simulink model "[LQG] Inverse_Pendulum_discretized"  (R2022b)
settings: Solver=ode4  StartTime=0.0  StopTime=50  FixedStep=0.005  RelTol=1e-3
values from neighbouring files (symbols this model uses):
  Ad = sys_d.A    [Inverse_Pendulum_parameters_discrete.m]
  b = 0.00007892    (= 7.892e-05)    [Inverse_Pendulum_parameters.m]    (also in Inverse_Pendulum_parameters_discrete.m; [LQG] Inverse_Pendulum_parameters.m; [LQR] Inverse_Pendulum_parameters.m)
  Bd = sys_d.B    [Inverse_Pendulum_parameters_discrete.m]
  c = 0.63    [Inverse_Pendulum_parameters.m]    (also in Inverse_Pendulum_parameters_discrete.m; [LQG] Inverse_Pendulum_parameters.m; [LQR] Inverse_Pendulum_parameters.m)
  Cd = sys_d.C    [Inverse_Pendulum_parameters_discrete.m]
  g = 9.81    [Inverse_Pendulum_parameters.m]    (also in Inverse_Pendulum_parameters_discrete.m; [LQG] Inverse_Pendulum_parameters.m; [LQR] Inverse_Pendulum_parameters.m)
  J = 0.0007176    [Inverse_Pendulum_parameters.m]    (also in Inverse_Pendulum_parameters_discrete.m = 0.000596; [LQG] Inverse_Pendulum_parameters.m; [LQR] Inverse_Pendulum_parameters.m)
  k_swing = 12    [Inverse_Pendulum_parameters.m]    (also in Inverse_Pendulum_parameters_discrete.m = 42; [LQG] Inverse_Pendulum_parameters.m; [LQR] Inverse_Pendulum_parameters.m)
  kb = 0.031    [Inverse_Pendulum_parameters.m]    (also in Inverse_Pendulum_parameters_discrete.m; [LQG] Inverse_Pendulum_parameters.m; [LQR] Inverse_Pendulum_parameters.m)
  Kd = dlqr(Ad, Bd, Q, R)    [Inverse_Pendulum_parameters_discrete.m]
  Kkd = dlqe(Ad, G, Cd, Qn, Rn)    [Inverse_Pendulum_parameters_discrete.m]
  kt = 0.031    [Inverse_Pendulum_parameters.m]    (also in Inverse_Pendulum_parameters_discrete.m; [LQG] Inverse_Pendulum_parameters.m; [LQR] Inverse_Pendulum_parameters.m)
  l = 0.2    [Inverse_Pendulum_parameters.m]    (also in Inverse_Pendulum_parameters_discrete.m = 0.1; [LQG] Inverse_Pendulum_parameters.m; [LQR] Inverse_Pendulum_parameters.m)
  M = 0.136    [Inverse_Pendulum_parameters.m]    (also in Inverse_Pendulum_parameters_discrete.m = 0.1; [LQG] Inverse_Pendulum_parameters.m; [LQR] Inverse_Pendulum_parameters.m)
  m = 0.1    [Inverse_Pendulum_parameters.m]    (also in Inverse_Pendulum_parameters_discrete.m = 0.04467; [LQG] Inverse_Pendulum_parameters.m; [LQR] Inverse_Pendulum_parameters.m)
  r = 0.006    [Inverse_Pendulum_parameters.m]    (also in Inverse_Pendulum_parameters_discrete.m; [LQG] Inverse_Pendulum_parameters.m; [LQR] Inverse_Pendulum_parameters.m)
  Rm = 12.5    [Inverse_Pendulum_parameters.m]    (also in Inverse_Pendulum_parameters_discrete.m; [LQG] Inverse_Pendulum_parameters.m; [LQR] Inverse_Pendulum_parameters.m)
  Ts = 0.005    [Inverse_Pendulum_parameters_discrete.m]
libraries: simulink x8, mpclib x2
settings Model: Creator=ADMIN  LastModifiedBy=ADMIN
settings OptimizationCC: DefaultParameterBehavior=Inlined  EnhancedBackFolding=on  PassReuseOutputArgsAs=Individual arguments  ZeroExternalMemoryAtStartup=off  ZeroInternalMemoryAtStartup=off  OptimizeBlockOrder=speed  DifferentSizesBufferReuse=on  OptimizationCustomize=off  EfficientTunableParamExpr=on
settings DebuggingCC: ParameterTunabilityLossMsg=error
settings SFSimCC: MATLABDynamicMemAlloc=off
settings RTWCC: Description=Embedded Coder  SystemTargetFile=ert.tlc  GenCodeOnly=on  TemplateMakefile=ert_default_tmf  GPUComputeCapability=5.0
settings CodeAppCC: ForceParamTrailComments=on  IgnoreCustomStorageClasses=off  OperatorAnnotations=on  SimulinkDataObjDesc=on  SFDataObjDesc=on  InsertBlockDesc=on
settings ERTTargetCC: TargetLangStandard=C99 (ISO)  GenerateSampleERTMain=on  InlinedParameterPlacement=NonHierarchical  ERTCustomFileTemplate=example_file_process.tlc

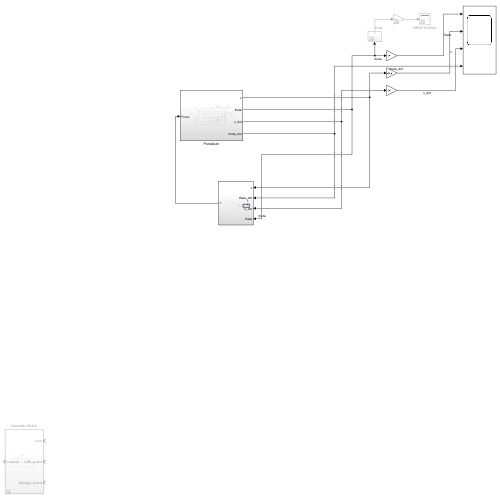
[thumbnail: Simulink's stored preview of the top-level diagram]
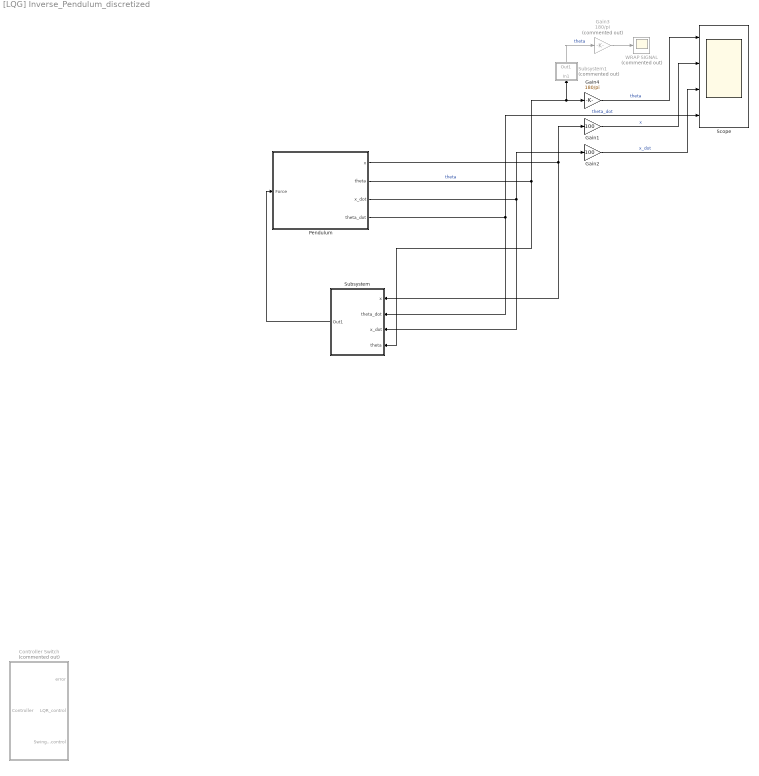
== system [LQG] Inverse_Pendulum_discretized ==
  Controller Switch : Subsystem  Commented=on
  Gain1 : Gain  Gain=100
  Gain2 : Gain  Gain=100
  Gain3 : Gain  Commented=on  Gain=180/pi
  Gain4 : Gain  Gain=180/pi
  Pendulum : Subsystem
  Scope : Scope  NumInputPorts=4
  Subsystem : Subsystem
  Subsystem1 : Subsystem  Commented=on
  WRAP SIGNAL : Scope  Commented=on
  wires:
  Pendulum/1(x) -> Gain1/1, Subsystem/1(x)
  Pendulum/3(x_dot) -> Gain2/1, Subsystem/3(x_dot)
  Pendulum/4(theta_dot) -> Scope/4, Subsystem/2(theta_dot)  "theta_dot"
  Gain1/1 -> Scope/2  "x"
  Gain2/1 -> Scope/3  "x_dot"
  Pendulum/2(theta) -> Subsystem/4(theta), Subsystem1/1(In1), Gain4/1  "theta"
  Gain3/1 -> WRAP SIGNAL/1
  Subsystem1/1(Out1) -> Gain3/1  "theta"
  Gain4/1 -> Scope/1  "theta"
  Subsystem/1(Out1) -> Pendulum/1(Force)

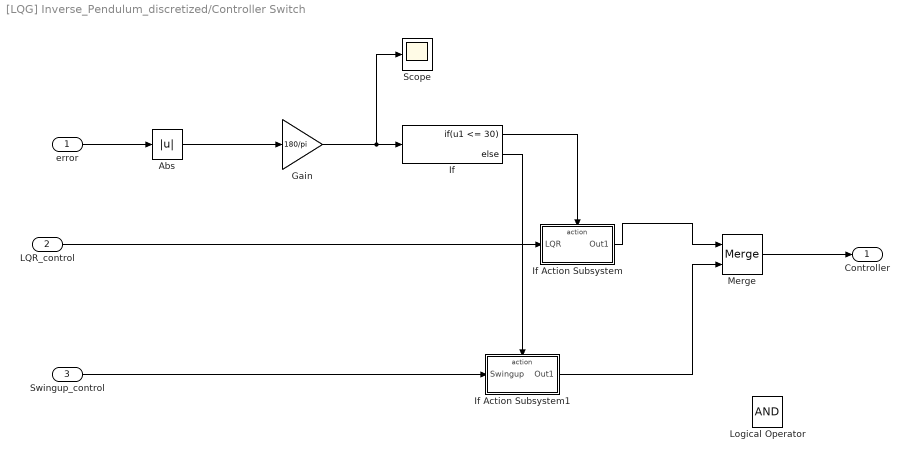
== system [LQG] Inverse_Pendulum_discretized/Controller Switch ==
  error : Inport
  LQR_control : Inport  Port=2
  Swingup_control : Inport  Port=3
  Abs : Abs  SaturateOnIntegerOverflow=off
  Gain : Gain  Gain=180/pi
  If : If  IfExpression=u1 <= 30
  If Action Subsystem : Subsystem  TreatAsAtomicUnit=on
  If Action Subsystem1 : Subsystem  TreatAsAtomicUnit=on
  Logical Operator : Logic  AllPortsSameDT=off  OutDataTypeStr=boolean
  Merge : Merge
  Scope : Scope
  Controller : Outport
  wires:
  error/1 -> Abs/1
  Abs/1 -> Gain/1
  Gain/1 -> Scope/1, If/1
  If/1 -> If Action Subsystem/Action
  LQR_control/1 -> If Action Subsystem/1(LQR)
  If/2 -> If Action Subsystem1/Action
  Swingup_control/1 -> If Action Subsystem1/1(Swingup)
  If Action Subsystem/1(Out1) -> Merge/1
  If Action Subsystem1/1(Out1) -> Merge/2
  Merge/1 -> Controller/1

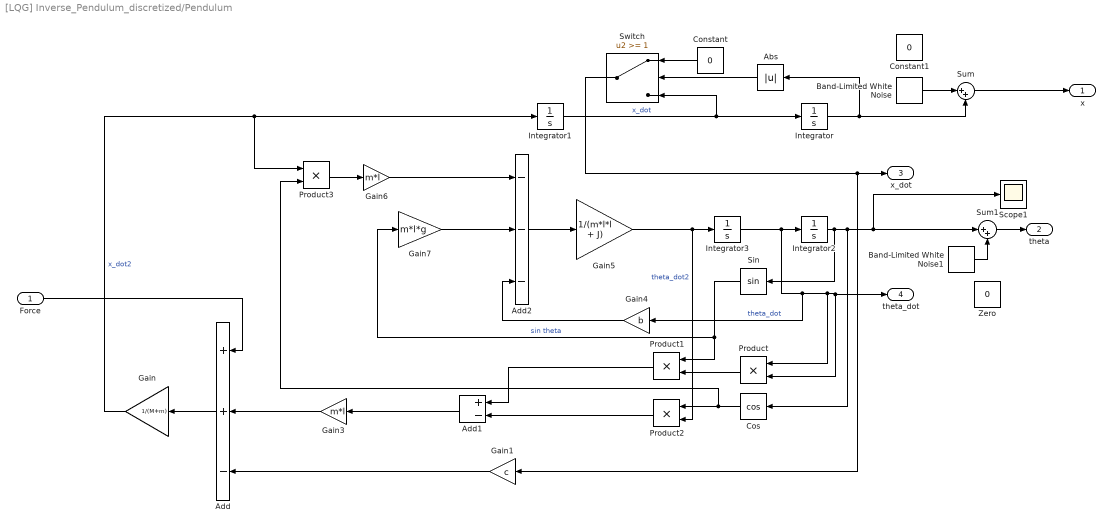
== system [LQG] Inverse_Pendulum_discretized/Pendulum ==
  Force : Inport
  Abs : Abs  SaturateOnIntegerOverflow=off
  Add : Sum  Inputs=++-
  Add1 : Sum  Inputs=+-
  Add2 : Sum  Inputs=---
  Band-Limited White Noise : simulink/Sources/Band-Limited White Noise  Cov=[0.000001]  Ts=0.1  seed=[23341]
  Band-Limited White Noise1 : simulink/Sources/Band-Limited White Noise  Cov=[0.000001]  Ts=0.1  seed=[23341]
  Constant : Constant  Value=0
  Constant1 : Constant  Value=0
  Cos : Trigonometry  Operator=cos
  Gain : Gain  Gain=1/(M+m)
  Gain1 : Gain  Gain=c
  Gain3 : Gain  Gain=m*l
  Gain4 : Gain  Gain=b
  Gain5 : Gain  Gain=1/(m*l*l + J)
  Gain6 : Gain  Gain=m*l
  Gain7 : Gain  Gain=m*l*g
  Integrator : Integrator  LimitOutput=on  UpperSaturationLimit=1  LowerSaturationLimit=-1
  Integrator1 : Integrator
  Integrator2 : Integrator
  Integrator3 : Integrator
  Product{,1..3} (4 alike) : Product
  Scope1 : Scope
  Sin : Trigonometry
  Sum : Sum  Inputs=|++
  Sum1 : Sum  Inputs=|++
  Switch : Switch  Threshold=1  SaturateOnIntegerOverflow=off  InputSameDT=off
  Zero : Constant  Value=0  OutDataTypeStr=Inherit: Inherit via back propagation
  x : Outport
  theta : Outport  Port=2
  x_dot : Outport  Port=3
  theta_dot : Outport  Port=4
  wires:
  Gain3/1 -> Add/2
  Integrator1/1 -> Switch/3, Integrator/1  "x_dot"
  Product/1 -> Product1/2
  Force/1 -> Add/1
  Product1/1 -> Add1/1
  Sin/1 -> Gain7/1, Product1/1  "sin theta"
  Gain6/1 -> Add2/1
  Add2/1 -> Gain5/1
  Integrator3/1 -> theta_dot/1, Product/2, Product/1, Gain4/1, Integrator2/1  "theta_dot"
  Gain5/1 -> Product2/2, Integrator3/1  "theta_dot2"
  Integrator2/1 -> Cos/1, Sum1/1, Scope1/1, Sin/1
  Add/1 -> Gain/1
  Gain/1 -> Product3/1, Integrator1/1  "x_dot2"
  Gain7/1 -> Add2/2
  Cos/1 -> Product3/2, Product2/1
  Product3/1 -> Gain6/1
  Gain4/1 -> Add2/3
  Product2/1 -> Add1/2
  Add1/1 -> Gain3/1
  Gain1/1 -> Add/3
  Sum/1 -> x/1
  Sum1/1 -> theta/1
  Abs/1 -> Switch/2
  Integrator/1 -> Abs/1, Sum/2
  Switch/1 -> Gain1/1, x_dot/1
  Constant/1 -> Switch/1
  Band-Limited White Noise/1 -> Sum/1
  Band-Limited White Noise1/1 -> Sum1/2

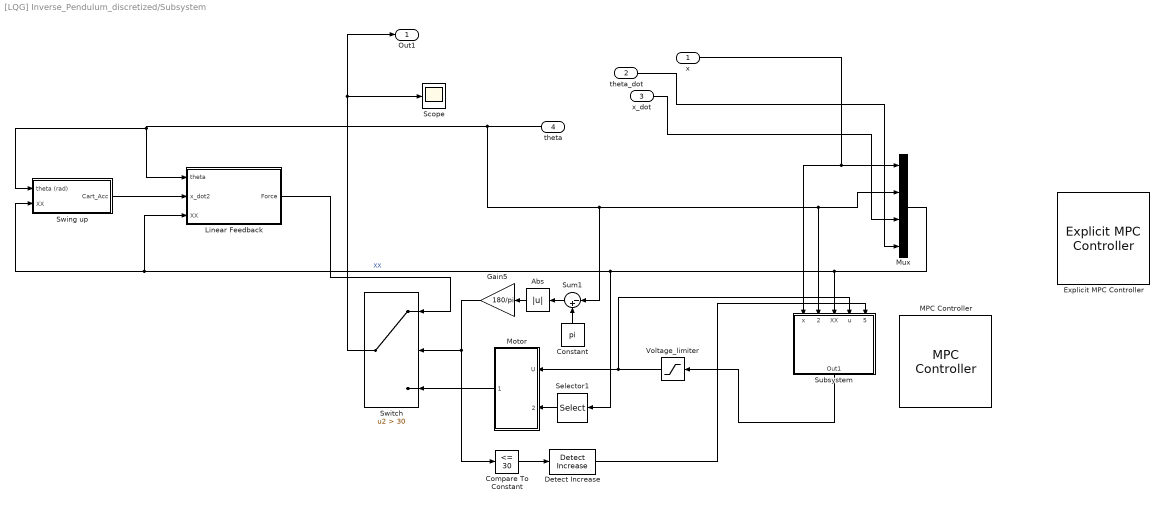
== system [LQG] Inverse_Pendulum_discretized/Subsystem ==
  x : Inport
  theta_dot : Inport  Port=2
  x_dot : Inport  Port=3
  theta : Inport  Port=4
  Abs : Abs  SaturateOnIntegerOverflow=off
  Compare To Constant : simulink/Logic and Bit Operations/Compare To Constant  relop=<=  const=30  OutDataTypeStr=boolean
  Constant : Constant  Value=pi
  Detect Increase : simulink/Logic and Bit Operations/Detect Increase  vinit=0.0  OutDataTypeStr=boolean
  Explicit MPC Controller : mpclib/Explicit MPC Controller  SCDEnableBlockLinearizationSpecification=on  is_multiple=0  enable_value=0  return_u0=off  md_inport=on  mv_inport=off  return_status=on  return_region=off  return_state=off  state_inport=off  BlockDataType=double  SampleTimeInherited=off  switch_inport=off
  Gain5 : Gain  Gain=180/pi
  Linear Feedback : Subsystem
  MPC Controller : mpclib/MPC Controller  SCDEnableBlockLinearizationSpecification=on  is_multiple=0  enable_value=0  return_u0=off  updateMPCinCallerWorkspace=on  md_inport=on  mv_inport=off  uref_inport=off  return_cost=off  return_mvseq=off  return_qpstatus=off  return_xseq=off  return_state=off  return_ovseq=off  state_inport=off  umin_inport=off  umax_inport=off  ymin_inport=off  ymax_inport=off  cc_inport=off  ywt_inport=off  uwt_inport=off  duwt_inport=off  rhoeps_inport=off  pm_inport=off  MaximumP=10  HorizonChoice=FixedHorizon  n_ts=1  n_p=10  n_mv=1  n_md=1  n_ud=0  n_mo=1  n_uo=0  BlockDataType=double  SampleTimeInherited=off  switch_inport=off
  Motor : Subsystem
  Mux : Mux
  Scope : Scope
  Selector1 : Selector  InputPortWidth=4  IndexOptions=Index vector (dialog)  Indices=3  OutputSizes=1
  Subsystem : Subsystem
  Sum1 : Sum  Inputs=|-+
  "Swing up " : Subsystem
  Switch : Switch  Criteria=u2 > Threshold  Threshold=30  SaturateOnIntegerOverflow=off  InputSameDT=off
  Voltage_limiter : Saturate  UpperLimit=12  LowerLimit=-12
  Out1 : Outport
  wires:
  theta/1 -> Mux/2, Subsystem/2(theta), Sum1/1, "Swing up "/1(theta (rad)), Linear Feedback/1(theta)
  Voltage_limiter/1 -> Subsystem/4(u), Motor/1(U)
  Selector1/1 -> Motor/2(x_dot)
  Compare To Constant/1 -> Detect Increase/1
  "Swing up "/1(Cart_Acc) -> Linear Feedback/2(x_dot2)
  Constant/1 -> Sum1/2
  Sum1/1 -> Abs/1
  Gain5/1 -> Compare To Constant/1, Switch/2
  Linear Feedback/1(Force) -> Switch/1
  Mux/1 -> Selector1/1, "Swing up "/2(XX), Linear Feedback/3(XX), Subsystem/3(XX)  "XX"
  Motor/1(Force) -> Switch/3
  Abs/1 -> Gain5/1
  Switch/1 -> Scope/1, Out1/1
  theta_dot/1 -> Mux/4
  x_dot/1 -> Mux/3
  x/1 -> Subsystem/1(x), Mux/1
  Detect Increase/1 -> Subsystem/5(Rising)
  Subsystem/1(Out1) -> Voltage_limiter/1

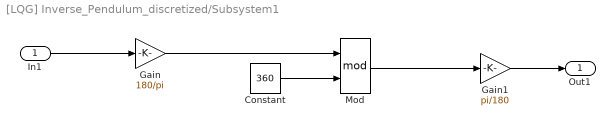
== system [LQG] Inverse_Pendulum_discretized/Subsystem1 ==
  In1 : Inport
  Constant : Constant  Value=360
  Gain : Gain  Gain=180/pi
  Gain1 : Gain  Gain=pi/180
  Mod : Math  Operator=mod
  Out1 : Outport
  wires:
  In1/1 -> Gain/1
  Constant/1 -> Mod/2
  Gain/1 -> Mod/1
  Mod/1 -> Gain1/1
  Gain1/1 -> Out1/1

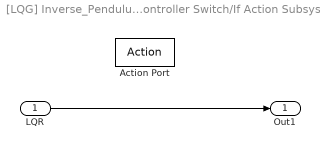
== system [LQG] Inverse_Pendulum_discretized/Controller Switch/If Action Subsystem ==
  LQR : Inport
  Action Port : ActionPort  ActionPortLabel=if(u1 <= 30)
  Out1 : Outport
  wires:
  LQR/1 -> Out1/1

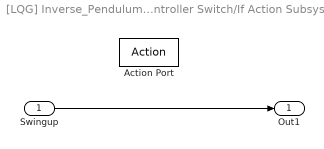
== system [LQG] Inverse_Pendulum_discretized/Controller Switch/If Action Subsystem1 ==
  Swingup : Inport
  Action Port : ActionPort  ActionPortLabel=else
  Out1 : Outport
  wires:
  Swingup/1 -> Out1/1

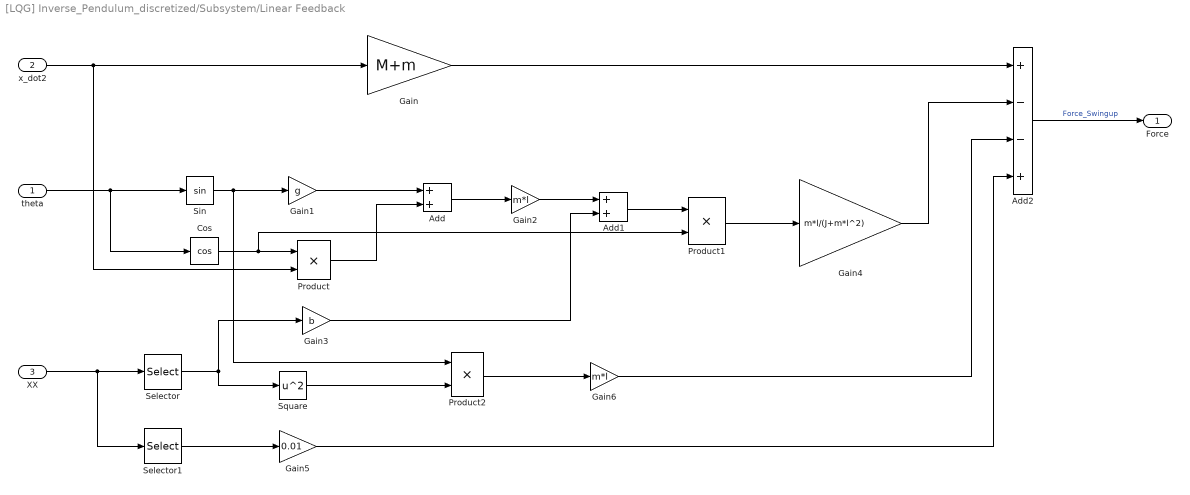
== system [LQG] Inverse_Pendulum_discretized/Subsystem/Linear Feedback ==
  theta : Inport
  x_dot2 : Inport  Port=2
  XX : Inport  Port=3
  Add : Sum
  Add1 : Sum
  Add2 : Sum  Inputs=+--+
  Cos : Trigonometry  Operator=cos
  Gain : Gain  Gain=M+m
  Gain1 : Gain  Gain=g
  Gain2 : Gain  Gain=m*l
  Gain3 : Gain  Gain=b
  Gain4 : Gain  Gain=m*l/(J+m*l^2)
  Gain5 : Gain  Gain=0.01
  Gain6 : Gain  Gain=m*l
  Product : Product
  Product1 : Product
  Product2 : Product
  Selector : Selector  InputPortWidth=4  IndexOptions=Index vector (dialog)  Indices=4  OutputSizes=1
  Selector1 : Selector  InputPortWidth=4  IndexOptions=Index vector (dialog)  Indices=3  OutputSizes=1
  Sin : Trigonometry
  Square : Math  Operator=square
  Force : Outport
  wires:
  theta/1 -> Cos/1, Sin/1
  x_dot2/1 -> Product/2, Gain/1
  Cos/1 -> Product1/2, Product/1
  Sin/1 -> Product2/1, Gain1/1
  Gain1/1 -> Add/1
  Product/1 -> Add/2
  Add/1 -> Gain2/1
  XX/1 -> Selector1/1, Selector/1
  Selector/1 -> Gain3/1, Square/1
  Gain2/1 -> Add1/1
  Gain3/1 -> Add1/2
  Add1/1 -> Product1/1
  Product1/1 -> Gain4/1
  Square/1 -> Product2/2
  Selector1/1 -> Gain5/1
  Product2/1 -> Gain6/1
  Gain6/1 -> Add2/3
  Gain4/1 -> Add2/2
  Gain/1 -> Add2/1
  Gain5/1 -> Add2/4
  Add2/1 -> Force/1  "Force_Swingup"

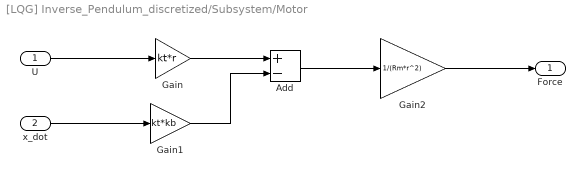
== system [LQG] Inverse_Pendulum_discretized/Subsystem/Motor ==
  U : Inport
  x_dot : Inport  Port=2
  Add : Sum  Inputs=+-
  Gain : Gain  Gain=kt*r
  Gain1 : Gain  Gain=kt*kb
  Gain2 : Gain  Gain=1/(Rm*r^2)
  Force : Outport
  wires:
  U/1 -> Gain/1
  x_dot/1 -> Gain1/1
  Gain/1 -> Add/1
  Gain1/1 -> Add/2
  Add/1 -> Gain2/1
  Gain2/1 -> Force/1

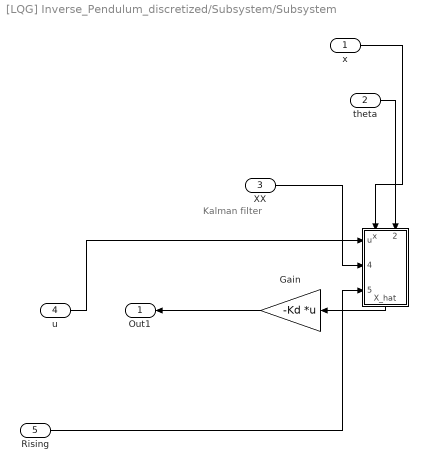
== system [LQG] Inverse_Pendulum_discretized/Subsystem/Subsystem ==
  note: Kalman filter
  x : Inport
  theta : Inport  Port=2
  XX : Inport  Port=3
  u : Inport  Port=4
  Rising : Inport  Port=5
  " " : Subsystem
      settings: PortSchema="{\"entries\":[{\"content\":{\"sides\":[{\"content\":{\"connectorIds\":[\"In1\",\"In2\"]},\"type\":\"ConnectorPlacement.EquallySpacedRectSide\",\"uuid\":\"213b765e-47fa-44cf-837a-76b4f9098c24\"},{\"content\":{\"connectorIds\":[\"Out1\"],\"side\":\"RIGHT\"},\"type\":\"ConnectorPlacement.EquallySpacedRectSide\",\"uuid\":\"45a7b12b-a4ed-4c45-ac3d-ce2c11d0f41c\"},{\"content\":{\"connectorIds\":[\"In3\",\"In4\",\"In5\"],\"side\":\"TOP\"},\"type\":\"ConnectorPlacement.EquallySpacedRectSide\",\"uuid\":\"3cd53e22-245a-4d13-9dac-306e9bf70ac5\"}]},\"type\":\"ConnectorPlacement.EquallySpacedConnector\",\"uuid\":\"c2a62d5e-615a-4291-9189-bd7e79077aeb\"}],\"packageUris\":[\"http://schema.mathworks.com/mf0/Connector/R2020b\"],\"version\":\"1.0\"}"
  Gain : Gain  Gain=-Kd  Multiplication=Matrix(K*u)
  Out1 : Outport
  wires:
  Rising/1 -> " "/5(Rising)
  theta/1 -> " "/2(theta)
  " "/1(X_hat) -> Gain/1
  x/1 -> " "/1(x)
  Gain/1 -> Out1/1
  u/1 -> " "/3(u)
  XX/1 -> " "/4(State)

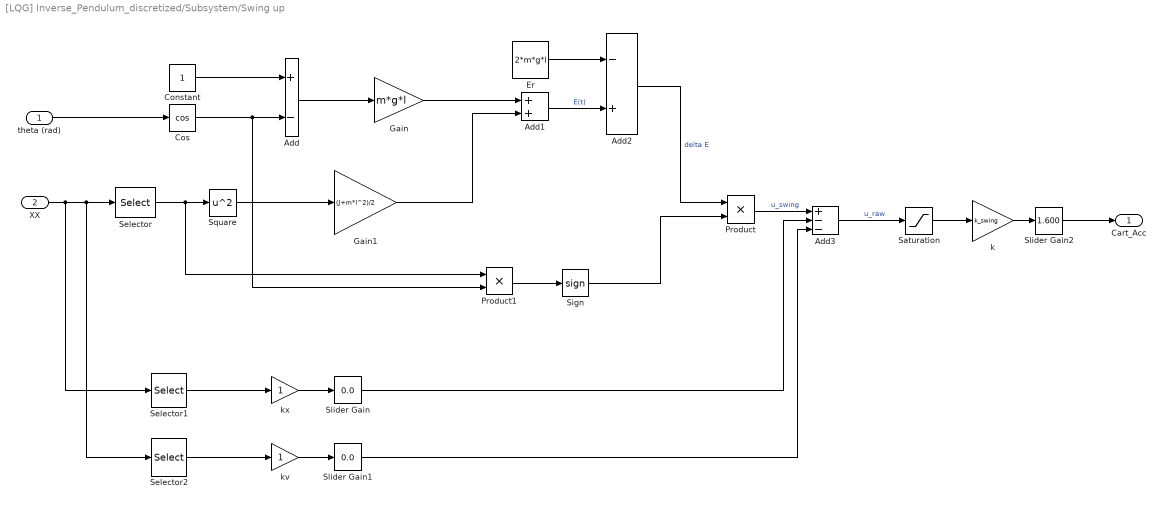
== system [LQG] Inverse_Pendulum_discretized/Subsystem/Swing up  ==
  theta (rad) : Inport
  XX : Inport  Port=2
  Add : Sum  Inputs=+-
  Add1 : Sum
  Add2 : Sum  Inputs=-+
  Add3 : Sum  Inputs=+--
  Constant : Constant
  Cos : Trigonometry  Operator=cos
  Er : Constant  Value=2*m*g*l
  Gain : Gain  Gain=m*g*l
  Gain1 : Gain  Gain=(J+m*l^2)/2
  Product : Product
  Product1 : Product
  Saturation : Saturate  UpperLimit=3*g  LowerLimit=-3*g
  Selector : Selector  InputPortWidth=4  IndexOptions=Index vector (dialog)  Indices=4  OutputSizes=1
  Selector1 : Selector  InputPortWidth=4  IndexOptions=Index vector (dialog)  Indices=1  OutputSizes=1
  Selector2 : Selector  InputPortWidth=4  IndexOptions=Index vector (dialog)  Indices=2  OutputSizes=1
  Sign : Signum
  Slider Gain : simulink/Math Operations/Slider Gain  gain=0.0  low=0  high=2
  Slider Gain1 : simulink/Math Operations/Slider Gain  gain=0.0  low=0  high=2
  Slider Gain2 : simulink/Math Operations/Slider Gain  gain=1.600  low=0  high=2
  Square : Math  Operator=square
  k : Gain  Gain=k_swing
  kv : Gain
  kx : Gain
  Cart_Acc : Outport
  wires:
  theta (rad)/1 -> Cos/1
  Cos/1 -> Product1/2, Add/2
  Constant/1 -> Add/1
  Add/1 -> Gain/1
  XX/1 -> Selector1/1, Selector2/1, Selector/1
  Selector/1 -> Product1/1, Square/1
  Gain/1 -> Add1/1
  Square/1 -> Gain1/1
  Gain1/1 -> Add1/2
  Add1/1 -> Add2/2  "E(t)"
  Er/1 -> Add2/1
  Add2/1 -> Product/1  "delta E"
  Sign/1 -> Product/2
  Product1/1 -> Sign/1
  Product/1 -> Add3/1  "u_swing"
  Slider Gain/1 -> Add3/2
  Selector1/1 -> kx/1
  kx/1 -> Slider Gain/1
  Selector2/1 -> kv/1
  kv/1 -> Slider Gain1/1
  Slider Gain1/1 -> Add3/3
  Add3/1 -> Saturation/1  "u_raw"
  k/1 -> Slider Gain2/1
  Slider Gain2/1 -> Cart_Acc/1
  Saturation/1 -> k/1

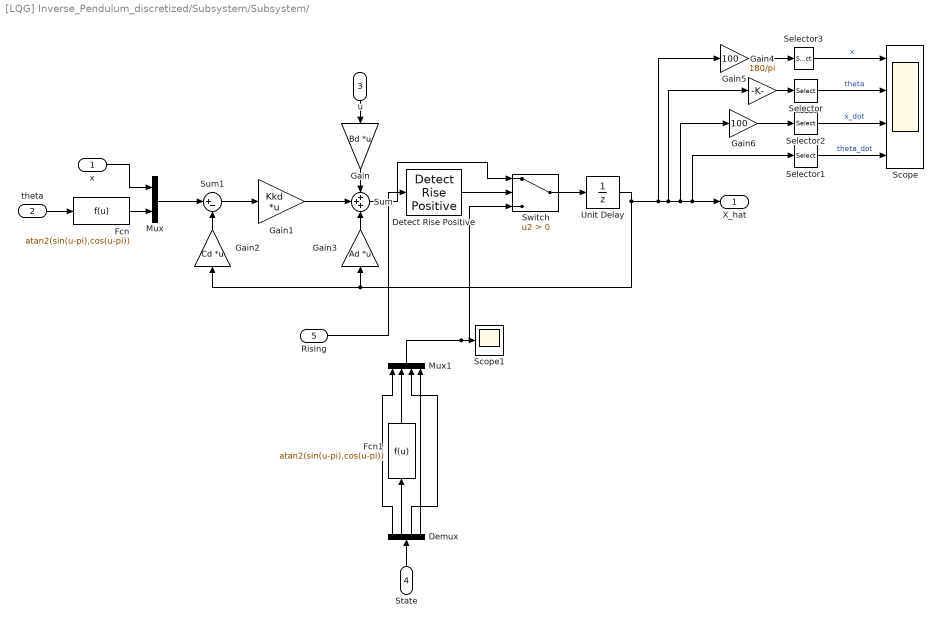
== system [LQG] Inverse_Pendulum_discretized/Subsystem/Subsystem/  ==
  x : Inport
  theta : Inport  Port=2
  u : Inport  Port=3
  State : Inport  Port=4
  Rising : Inport  Port=5
  Demux : Demux
  Detect Rise Positive : simulink/Logic and Bit Operations/Detect Rise Positive  vinit=0  OutDataTypeStr=boolean
  Fcn : Fcn  Expr=atan2(sin(u-pi),cos(u-pi))
  Fcn1 : Fcn  Expr=atan2(sin(u-pi),cos(u-pi))
  Gain : Gain  Gain=Bd  Multiplication=Matrix(K*u)
  Gain1 : Gain  Gain=Kkd  Multiplication=Matrix(K*u)
  Gain2 : Gain  Gain=Cd  Multiplication=Matrix(K*u)
  Gain3 : Gain  Gain=Ad  Multiplication=Matrix(K*u)
  Gain4 : Gain  Gain=180/pi
  Gain5 : Gain  Gain=100
  Gain6 : Gain  Gain=100
  Mux : Mux  Inputs=2
  Mux1 : Mux
  Scope : Scope  NumInputPorts=4
  Scope1 : Scope
  Selector : Selector  InputPortWidth=4  IndexOptions=Index vector (dialog)  Indices=2  OutputSizes=1
  Selector1 : Selector  InputPortWidth=4  IndexOptions=Index vector (dialog)  Indices=4  OutputSizes=1
  Selector2 : Selector  InputPortWidth=4  IndexOptions=Index vector (dialog)  Indices=3  OutputSizes=1
  Selector3 : Selector  InputPortWidth=4  IndexOptions=Index vector (dialog)  Indices=1  OutputSizes=1
  Sum : Sum  Inputs=+++
  Sum1 : Sum  Inputs=|+-
  Switch : Switch  Criteria=u2 > Threshold  SaturateOnIntegerOverflow=off  InputSameDT=off
  Unit Delay : UnitDelay  SampleTime=Ts  HasFrameUpgradeWarning=on
  X_hat : Outport
  wires:
  x/1 -> Mux/1
  Gain/1 -> Sum/1
  Sum1/1 -> Gain1/1
  Gain2/1 -> Sum1/2
  Gain1/1 -> Sum/2
  Gain3/1 -> Sum/3
  Unit Delay/1 -> Gain2/1, Gain3/1, Gain5/1, Gain4/1, Gain6/1, Selector1/1, X_hat/1
  u/1 -> Gain/1
  Mux/1 -> Sum1/1
  Selector/1 -> Scope/2  "theta"
  Selector1/1 -> Scope/4  "theta_dot"
  Selector2/1 -> Scope/3  "x_dot"
  Selector3/1 -> Scope/1  "x"
  Gain4/1 -> Selector/1
  Gain5/1 -> Selector3/1
  Gain6/1 -> Selector2/1
  theta/1 -> Fcn/1
  Fcn/1 -> Mux/2
  State/1 -> Demux/1
  Demux/2 -> Fcn1/1
  Fcn1/1 -> Mux1/2
  Demux/1 -> Mux1/1
  Demux/3 -> Mux1/3
  Demux/4 -> Mux1/4
  Mux1/1 -> Switch/3, Scope1/1
  Sum/1 -> Switch/1
  Rising/1 -> Detect Rise Positive/1
  Switch/1 -> Unit Delay/1
  Detect Rise Positive/1 -> Switch/2
